simulink model "MDL2_Longitudinal_Vehicle_Model_Mask"  (R2025b)
settings: Solver=VariableStepAuto  StartTime=0.0  StopTime=20  MaxStep=1/100  MinStep=1/1000  RelTol=1e-3
InitFcn:
  | mdl2_longitudinal_vehicle_init_params
undefined symbols (not defined in the file): F_T, m
settings Model: Creator=rkash  LastModifiedBy=rkash

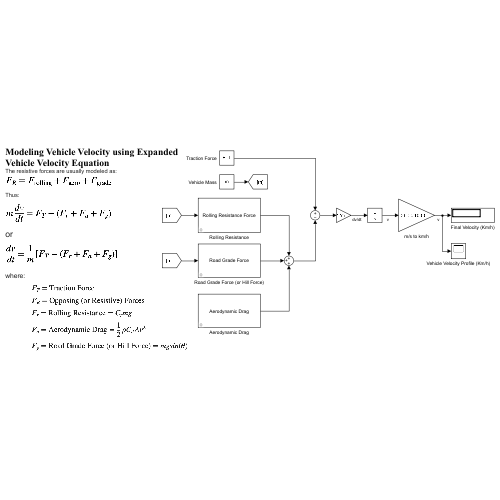
[thumbnail: Simulink's stored preview of the top-level diagram]
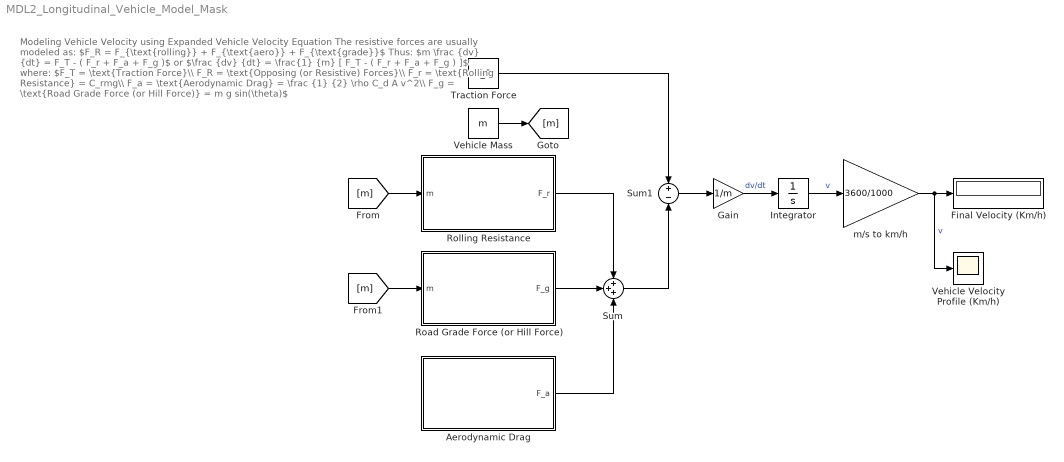
== system MDL2_Longitudinal_Vehicle_Model_Mask ==
  note: Modeling Vehicle Velocity using Expanded Vehicle Velocity Equation
      | The resistive forces are usually modeled as:
      | $F_R = F_{\text{rolling}} + F_{\text{aero}} + F_{\text{grade}}$
      | Thus:
      | $m \frac {dv} {dt} = F_T - ( F_r + F_a + F_g )$
      | or
      | $\frac {dv} {dt} = \frac{1} {m} [ F_T - ( F_r + F_a + F_g ) ]$
      | where:
      | $F_T = \text{Traction Force}\\ F_R = \text{Opposing (or Resistive) Forces}\\ F_r = \text{Rolling Resistance} = C_rmg\\ F_a = \text{Aerodynamic Drag} = \frac {1} {2} \rho C_d A v^2\\ F_g = \text{Road Grade Force (or Hill Force)} = m g sin(\theta)$
  Aerodynamic Drag : Subsystem  mask(Aerodynamic Drag Force){rho=1.225, C_d=0.32, A=2.2, v=20}
      mask prompts: rho "Air Density (kg/m^3)"; C_d "Drag Coefficient"; A "Vehicle Frontal Area (m^2)"; v "Vehicle Velocity Relative to Air (m/s)"
      mask help:
      | This subsystem computes the aerodynamic drag force.
      |
      | It computes the expression:
      |
      | (1/2) .* rho .* Cd .* A .* (v .^ 2)
      |
      | Where,
      |
      | rho is Air Density (kg/m^3)
      | Cd is Drag Coefficient (constant)
      | A is Vehicle Frontal Area (m^2)
      | v is Vehicle Velocity Relative to Air (m/s)v
      mask TypeOptions rho: Air Density/Value
      mask TypeOptions C_d: Drag Coefficient/Value
      mask TypeOptions A: Vehicle Frontal Area/Value
      mask TypeOptions v: Vehicle Velocity Relative to Air/Value
      mask Display: disp('Aerodynamic Drag');
  Final Velocity (Km/h) : Display
  Gain : Gain  Gain=1/m
  Integrator : Integrator
  Road Grade Force (or Hill Force) : Subsystem  mask(Road Grade Force){g=9.81, theta=0}
      mask prompts: g "Gravitational Acceleration (m/s^2)"; theta "Road Slope Angle (radians)"
      mask help:
      | This subsystem computes the road grade force (or hill force).
      |
      | It computes the expression:
      |
      | m .* g  .* sin(theta)
      |
      | Where,
      |
      | m is Mass of the Vehicle (kg)
      | g is Gravitational Acceleration = 9.81 m/s^2
      | theta is Road Slope Angle (radians)
      mask TypeOptions g: Gravitational Acceleration/Value
      mask TypeOptions theta: Road Slope Angle/Value
      mask Display: disp('Road Grade Force');
  Rolling Resistance : Subsystem  mask(Rolling Resistance Force){g=9.81, C_r=0.015}
      mask prompts: g "Gravitational Acceleration (m/s^2)"; C_r "Rolling Coefficient"
      mask help:
      | This subsystem computes the rolling resistance force.
      |
      | It computes the equation:
      |
      | Cr .* m .* g
      |
      | Where,
      |
      | Cr is Rolling Resistance Coefficient (constant)
      | m is Mass of the Vehicle (kg)
      | g is Gravitational Acceleration = 9.81 m/s^2
      mask TypeOptions g: Gravitational Acceleration/Value
      mask TypeOptions C_r: Rolling Coefficient/Value
      mask Display: disp('Rolling Resistance Force');
  Sum : Sum  Inputs=+++
  Sum1 : Sum  Inputs=+-
  Traction Force : Constant  Value=F_T
  Vehicle Mass : Constant  Value=m
  Vehicle Velocity Profile (Km/h) : Scope
      settings: ActiveDisplayYMinimum=-1  ActiveDisplayYMaximum=1
  m/s to km/h : Gain  Gain=3600/1000
  wires:
  Rolling Resistance/1(F_r) -> Sum/1
  Road Grade Force (or Hill Force)/1(F_g) -> Sum/2
  Aerodynamic Drag/1(F_a) -> Sum/3
  Traction Force/1 -> Sum1/1
  Sum/1 -> Sum1/2
  Sum1/1 -> Gain/1
  Gain/1 -> Integrator/1  "dv/dt"
  Integrator/1 -> m/s to km/h/1  "v"
  m/s to km/h/1 -> Vehicle Velocity Profile (Km/h)/1, Final Velocity (Km/h)/1  "v"
  Vehicle Mass/1 -> [m]
  [m] -> Rolling Resistance/1(m)
  [m] -> Road Grade Force (or Hill Force)/1(m)

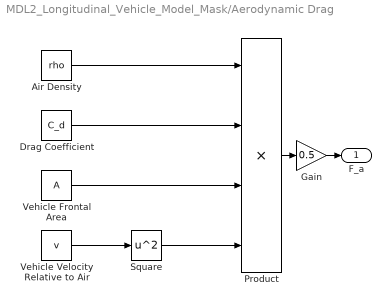
== system MDL2_Longitudinal_Vehicle_Model_Mask/Aerodynamic Drag ==
  Air Density : Constant  Value=rho
  Drag Coefficient : Constant  Value=C_d
  Gain : Gain  Gain=0.5
  Product : Product  Inputs=4
  Square : Math  Operator=square
  Vehicle Frontal Area : Constant  Value=A
  Vehicle Velocity Relative to Air : Constant  Value=v
  F_a : Outport
  wires:
  Vehicle Frontal Area/1 -> Product/3
  Drag Coefficient/1 -> Product/2
  Air Density/1 -> Product/1
  Product/1 -> Gain/1
  Gain/1 -> F_a/1
  Vehicle Velocity Relative to Air/1 -> Square/1
  Square/1 -> Product/4

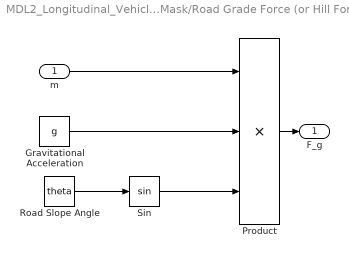
== system MDL2_Longitudinal_Vehicle_Model_Mask/Road Grade Force (or Hill Force) ==
  m : Inport
  Gravitational Acceleration : Constant  Value=g
  Product : Product  Inputs=3
  Road Slope Angle : Constant  Value=theta
  Sin : Trigonometry
  F_g : Outport
  wires:
  m/1 -> Product/1
  Gravitational Acceleration/1 -> Product/2
  Product/1 -> F_g/1
  Sin/1 -> Product/3
  Road Slope Angle/1 -> Sin/1

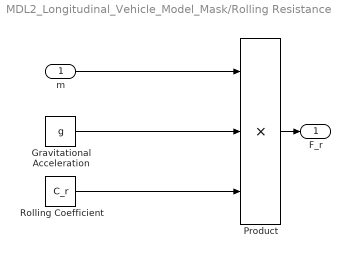
== system MDL2_Longitudinal_Vehicle_Model_Mask/Rolling Resistance ==
  m : Inport
  Gravitational Acceleration : Constant  Value=g
  Product : Product  Inputs=3
  Rolling Coefficient : Constant  Value=C_r
  F_r : Outport
  wires:
  Rolling Coefficient/1 -> Product/3
  Product/1 -> F_r/1
  Gravitational Acceleration/1 -> Product/2
  m/1 -> Product/1
